simulink model "G_analog"  (R2020b)
settings: Solver=VariableStepAuto  StartTime=0.0  StopTime=10.0  RelTol=1e-3
libraries: cstblocks x8
settings Model: Creator=jasper  LastModifiedBy=jasper

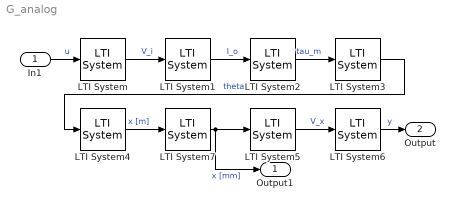
== system G_analog ==
  In1 : Inport
  LTI System : cstblocks/LTI System  sys=K_dac  IC=[]
  LTI System1 : cstblocks/LTI System  sys=G_amp  IC=[]
  LTI System2 : cstblocks/LTI System  sys=K_t  IC=[]
  LTI System3 : cstblocks/LTI System  sys=G_m  IC=[]
  LTI System4 : cstblocks/LTI System  sys=r  IC=[]
  LTI System5 : cstblocks/LTI System  sys=K_lvdt  IC=[]
  LTI System6 : cstblocks/LTI System  sys=K_adc  IC=[]
  LTI System7 : cstblocks/LTI System  sys=1000  IC=[]
  Output1 : Outport
  Output : Outport  Port=2
  wires:
  LTI System/1 -> LTI System1/1  "V_i"
  LTI System1/1 -> LTI System2/1  "I_o"
  LTI System2/1 -> LTI System3/1  "tau_m"
  LTI System3/1 -> LTI System4/1  "theta"
  LTI System4/1 -> LTI System7/1  "x [m]"
  LTI System5/1 -> LTI System6/1  "V_x"
  In1/1 -> LTI System/1  "u"
  LTI System6/1 -> Output/1  "y"
  LTI System7/1 -> Output1/1, LTI System5/1  "x [mm]"
